simulink model "model"  (R2019a)
settings: Solver=ode113  StartTime=0.0  StopTime=25  RelTol=1e-3
undefined symbols (not defined in the file): sigbuilder_block
libraries: simulink x3
settings Model: Creator=lenovo  LastModifiedBy=FF
settings DataIOCC: ReturnWorkspaceOutputs=off
settings DebuggingCC: ArithmeticOperatorsInVariantConditions=warning
settings SFSimCC: SimUseLocalCustomCode=off
settings RTWCC: RTWUseLocalCustomCode=off

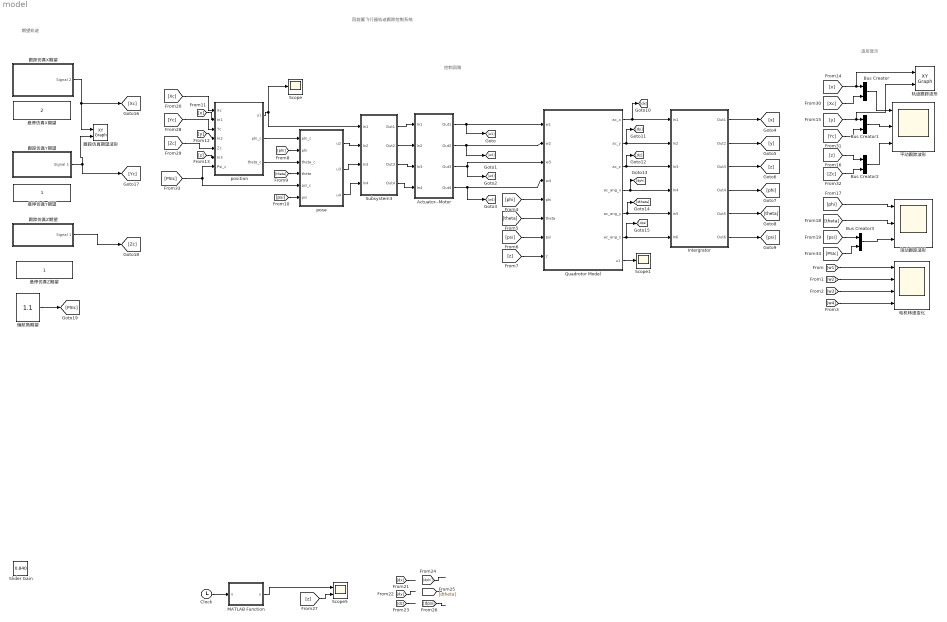
== system model ==
  note: 波形显示
  note: 控制回路
  note: 期望轨迹
  note: 四旋翼飞行器轨迹跟踪控制系统
  Actuator--Motor : Subsystem
  Bus Creator{,1..3} (4 alike) : BusCreator  Inputs=2
  Clock : Clock
  Intergrator : Subsystem
  MATLAB Function : MATLAB Function  TreatAsAtomicUnit=on
  Quadrotor Model : MATLAB Function  TreatAsAtomicUnit=on
  Scope : Scope
  Scope1 : Scope
  Scope5 : Scope  NumInputPorts=2
  Slider Gain : simulink/Math Operations/Slider Gain  gain=0.840  low=0  high=2
  Subsystem3 : Subsystem
  pose : Subsystem
  position : Subsystem
  偏航角期望 : Constant  Value=1.1
  平动跟踪波形 : Scope  NumInputPorts=3
  悬停仿真X期望 : Constant  Value=2
  悬停仿真Y期望 : Constant
  悬停仿真Z期望 : Constant
  滚动跟踪波形 : Scope  NumInputPorts=3
  电机转速变化 : Scope  NumInputPorts=4
  跟踪仿真X期望 : Subsystem  Tag=STV Subsys  LoadFcn=sigbuilder_block('load');  StartFcn=sigbuilder_block('start');  StopFcn=sigbuilder_block('stop');  ClipboardFcn=sigbuilder_block('clipboard');  mask(Sigbuilder block){tuvar=[0:10]}
      mask help: Simulink:masks:SigbuilderBlock_MD
      mask init:
      | if ~strcmp(get_param(bdroot(gcbh),'SimulationStatus'),'stopped') tuvar = sigbuilder_block('maskInit'); end
      settings: CopyFcn=sigbuilder_block('copy');  DeleteFcn=sigbuilder_block('delete');  ModelCloseFcn=sigbuilder_block('modelClose');  PreSaveFcn=sigbuilder_block('preSave');  PauseFcn=sigbuilder_block('pause');  ContinueFcn=sigbuilder_block('continue');  NameChangeFcn=sigbuilder_block('namechange');  OpenFcn=sigbuilder_block('open',[374.4 110.4 550.8 400.2 ]);  CloseFcn=sigbuilder_block('close');
      mask Display: plot(0, 0, 100, 100,[2, 2, 32, 32, 2], [68, 8, 8, 68, 68],[32, 2], [38, 38], [32, 19, 2],[53, 60, 44], [32, 17, 17, 2],[16, 16, 31, 31]);txt = getActiveGroup(gcbh);text(2, 100, txt,'verticalAlignment', 'top');
  跟踪仿真Y期望 : Subsystem  Tag=STV Subsys  LoadFcn=sigbuilder_block('load');  StartFcn=sigbuilder_block('start');  StopFcn=sigbuilder_block('stop');  ClipboardFcn=sigbuilder_block('clipboard');  mask(Sigbuilder block){tuvar=[0:10]}
      mask help: Simulink:masks:SigbuilderBlock_MD
      mask init:
      | if ~strcmp(get_param(bdroot(gcbh),'SimulationStatus'),'stopped') tuvar = sigbuilder_block('maskInit'); end
      settings: CopyFcn=sigbuilder_block('copy');  DeleteFcn=sigbuilder_block('delete');  ModelCloseFcn=sigbuilder_block('modelClose');  PreSaveFcn=sigbuilder_block('preSave');  PauseFcn=sigbuilder_block('pause');  ContinueFcn=sigbuilder_block('continue');  NameChangeFcn=sigbuilder_block('namechange');  OpenFcn=sigbuilder_block('open',[268.8 123 550.8 400.2 ]);  CloseFcn=sigbuilder_block('close');
      mask Display: plot(0, 0, 100, 100,[2, 2, 32, 32, 2], [68, 8, 8, 68, 68],[32, 2], [38, 38], [32, 19, 2],[53, 60, 44], [32, 17, 17, 2],[16, 16, 31, 31]);txt = getActiveGroup(gcbh);text(2, 100, txt,'verticalAlignment', 'top');
  跟踪仿真Z期望 : Subsystem  Tag=STV Subsys  LoadFcn=sigbuilder_block('load');  StartFcn=sigbuilder_block('start');  StopFcn=sigbuilder_block('stop');  ClipboardFcn=sigbuilder_block('clipboard');  mask(Sigbuilder block){tuvar=[0:10]}
      mask help: Simulink:masks:SigbuilderBlock_MD
      mask init:
      | if ~strcmp(get_param(bdroot(gcbh),'SimulationStatus'),'stopped') tuvar = sigbuilder_block('maskInit'); end
      settings: CopyFcn=sigbuilder_block('copy');  DeleteFcn=sigbuilder_block('delete');  ModelCloseFcn=sigbuilder_block('modelClose');  PreSaveFcn=sigbuilder_block('preSave');  PauseFcn=sigbuilder_block('pause');  ContinueFcn=sigbuilder_block('continue');  NameChangeFcn=sigbuilder_block('namechange');  OpenFcn=sigbuilder_block('open',[359.4 96 550.8 400.2 ]);  CloseFcn=sigbuilder_block('close');
      mask Display: plot(0, 0, 100, 100,[2, 2, 32, 32, 2], [68, 8, 8, 68, 68],[32, 2], [38, 38], [32, 19, 2],[53, 60, 44], [32, 17, 17, 2],[16, 16, 31, 31]);txt = getActiveGroup(gcbh);text(2, 100, txt,'verticalAlignment', 'top');
  跟踪仿真期望波形 : simulink/Sinks/XY Graph  xmin=0  xmax=3  ymin=0  ymax=3  st=1
  轨迹跟踪波形 : simulink/Sinks/XY Graph  xmin=0  xmax=3  ymin=0  ymax=3  st=7.5
  wires:
  Quadrotor Model/2(ac_y) -> Intergrator/2(In2), [dy]
  Quadrotor Model/4(ac_ang_x) -> Intergrator/4(In4), [dphi]
  Quadrotor Model/5(ac_ang_y) -> Intergrator/5(In5), [dtheta]
  Quadrotor Model/6(ac_ang_z) -> Intergrator/6(In6), [dpsi]
  Clock/1 -> MATLAB Function/1(u)
  Actuator--Motor/1(Out1) -> Quadrotor Model/1(w1), [w1]
  Actuator--Motor/2(Out2) -> [w2], Quadrotor Model/2(w2)
  Actuator--Motor/3(Out3) -> [w3], Quadrotor Model/3(w3)
  Actuator--Motor/4(Out4) -> Quadrotor Model/4(w4), [w4]
  pose/3(u4) -> Subsystem3/4(In4)
  pose/2(u3) -> Subsystem3/3(In3)
  pose/1(u2) -> Subsystem3/2(In2)
  position/1(u1) -> Scope/1, Subsystem3/1(In1)
  position/3(theta_c) -> pose/3(theta_c)
  position/2(phi_c) -> pose/1(phi_c)
  Quadrotor Model/7(u1) -> Scope1/1
  Subsystem3/1(Out1) -> Actuator--Motor/1(In1)
  Subsystem3/2(Out2) -> Actuator--Motor/2(In2)
  Subsystem3/3(Out3) -> Actuator--Motor/3(In3)
  Subsystem3/4(Out4) -> Actuator--Motor/4(In4)
  Quadrotor Model/1(ac_x) -> Intergrator/1(In1), [dx]
  Quadrotor Model/3(ac_z) -> Intergrator/3(In3), [dz]
  [w1] -> 电机转速变化/1
  [w2] -> 电机转速变化/2
  [w3] -> 电机转速变化/3
  [w4] -> 电机转速变化/4
  Intergrator/1(Out1) -> [x]
  Intergrator/2(Out2) -> [y]
  Intergrator/4(Out4) -> [phi]
  Intergrator/5(Out5) -> [theta]
  Intergrator/6(Out6) -> [psi]
  [phi] -> Quadrotor Model/5(phi)
  [theta] -> Quadrotor Model/6(theta)
  [psi] -> Quadrotor Model/7(psi)
  [z] -> Quadrotor Model/8(z)
  Intergrator/3(Out3) -> [z]
  [phi] -> pose/2(phi)
  [theta] -> pose/4(theta)
  [psi] -> pose/6(psi)
  [x] -> position/2(In1)
  [y] -> position/4(In2)
  [z] -> position/6(In3)
  [x] -> 轨迹跟踪波形/1, Bus Creator/1
  [y] -> Bus Creator1/1, 轨迹跟踪波形/2
  [phi] -> 滚动跟踪波形/1
  [theta] -> 滚动跟踪波形/2
  MATLAB Function/1(y) -> Scope5/1
  [dx] -> ?
  [dy] -> ?
  [dz] -> ?
  [dphi] -> ?
  [dtheta] -> ?
  [dpsi] -> ?
  [z] -> Scope5/2
  跟踪仿真X期望/1(Signal 2) -> 跟踪仿真期望波形/1, [Xc]
  跟踪仿真Y期望/1(Signal 1) -> [Yc], 跟踪仿真期望波形/2
  [Xc] -> position/1(Xc)
  [Yc] -> position/3(Yc)
  [Zc] -> position/5(Zc)
  [Xc] -> Bus Creator/2
  Bus Creator/1 -> 平动跟踪波形/1
  [Yc] -> Bus Creator1/2
  Bus Creator1/1 -> 平动跟踪波形/2
  [z] -> Bus Creator2/1
  [Zc] -> Bus Creator2/2
  Bus Creator2/1 -> 平动跟踪波形/3
  偏航角期望/1 -> [PSIc]
  [PSIc] -> position/7(Psi_c), pose/5(psi_c)
  [psi] -> Bus Creator3/1
  [PSIc] -> Bus Creator3/2
  Bus Creator3/1 -> 滚动跟踪波形/3
  跟踪仿真Z期望/1(Signal 1) -> [Zc]

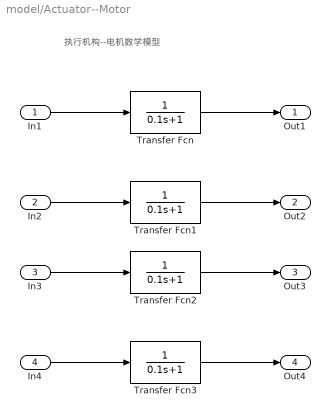
== system model/Actuator--Motor ==
  note: 执行机构--电机数学模型
  In1 : Inport
  In2 : Inport  Port=2
  In3 : Inport  Port=3
  In4 : Inport  Port=4
  Transfer Fcn{,1..3} (4 alike) : TransferFcn  Denominator=[0.1 1]
  Out1 : Outport
  Out2 : Outport  Port=2
  Out3 : Outport  Port=3
  Out4 : Outport  Port=4
  wires:
  In1/1 -> Transfer Fcn/1
  In2/1 -> Transfer Fcn1/1
  In3/1 -> Transfer Fcn2/1
  In4/1 -> Transfer Fcn3/1
  Transfer Fcn/1 -> Out1/1
  Transfer Fcn1/1 -> Out2/1
  Transfer Fcn2/1 -> Out3/1
  Transfer Fcn3/1 -> Out4/1

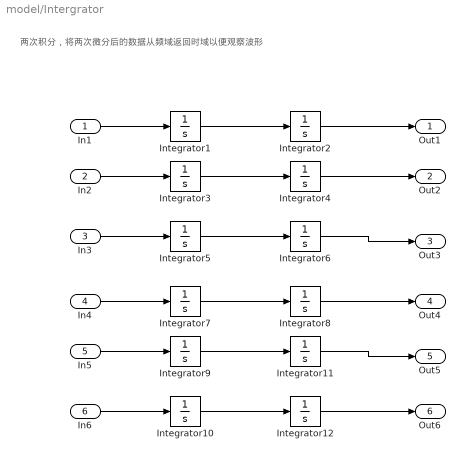
== system model/Intergrator ==
  note: 两次积分，将两次微分后的数据从频域返回时域以便观察波形
  In1 : Inport
  In2 : Inport  Port=2
  In3 : Inport  Port=3
  In4 : Inport  Port=4
  In5 : Inport  Port=5
  In6 : Inport  Port=6
  Integrator{1..12} (12 alike) : Integrator
  Out1 : Outport
  Out2 : Outport  Port=2
  Out3 : Outport  Port=3
  Out4 : Outport  Port=4
  Out5 : Outport  Port=5
  Out6 : Outport  Port=6
  wires:
  Integrator1/1 -> Integrator2/1
  Integrator2/1 -> Out1/1
  In1/1 -> Integrator1/1
  In2/1 -> Integrator3/1
  Integrator3/1 -> Integrator4/1
  Integrator4/1 -> Out2/1
  In3/1 -> Integrator5/1
  Integrator5/1 -> Integrator6/1
  Integrator8/1 -> Out4/1
  Integrator7/1 -> Integrator8/1
  In4/1 -> Integrator7/1
  Integrator11/1 -> Out5/1
  Integrator9/1 -> Integrator11/1
  In5/1 -> Integrator9/1
  Integrator12/1 -> Out6/1
  Integrator10/1 -> Integrator12/1
  In6/1 -> Integrator10/1
  Integrator6/1 -> Out3/1

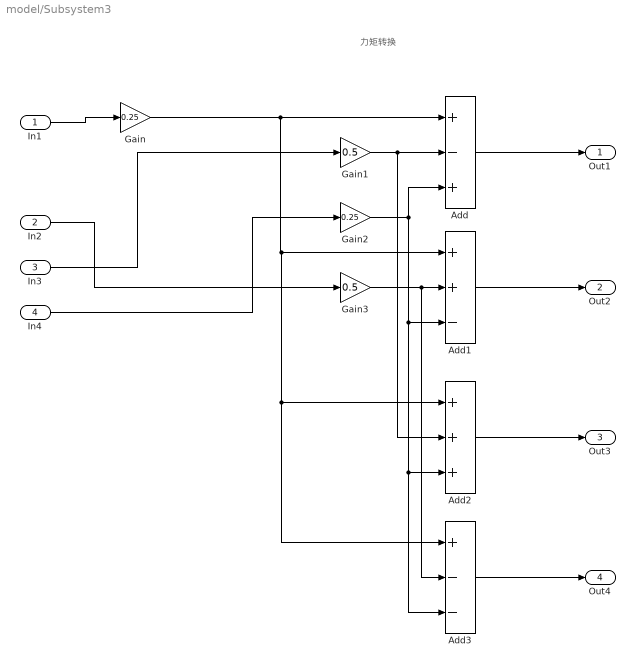
== system model/Subsystem3 ==
  note: 力矩转换
  In1 : Inport
  In2 : Inport  Port=2
  In3 : Inport  Port=3
  In4 : Inport  Port=4
  Add : Sum  Inputs=+-+
  Add1 : Sum  Inputs=++-
  Add2 : Sum  Inputs=+++
  Add3 : Sum  Inputs=+--
  Gain : Gain  Gain=0.25
  Gain1 : Gain  Gain=0.5
  Gain2 : Gain  Gain=0.25
  Gain3 : Gain  Gain=0.5
  Out1 : Outport
  Out2 : Outport  Port=2
  Out3 : Outport  Port=3
  Out4 : Outport  Port=4
  wires:
  In1/1 -> Gain/1
  In2/1 -> Gain3/1
  In4/1 -> Gain2/1
  Add3/1 -> Out4/1
  Add/1 -> Out1/1
  In3/1 -> Gain1/1
  Gain1/1 -> Add2/2, Add/2
  Add2/1 -> Out3/1
  Gain2/1 -> Add/3, Add2/3, Add3/3, Add1/3
  Gain3/1 -> Add3/2, Add1/2
  Add1/1 -> Out2/1
  Gain/1 -> Add3/1, Add2/1, Add1/1, Add/1

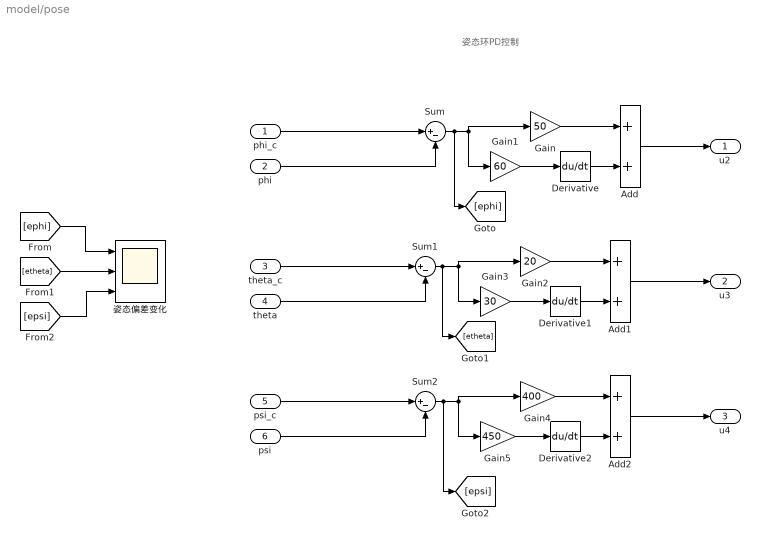
== system model/pose ==
  note: 姿态环PD控制
  phi_c : Inport
  phi : Inport  Port=2
  theta_c : Inport  Port=3
  theta : Inport  Port=4
  psi_c : Inport  Port=5
  psi : Inport  Port=6
  Add : Sum
  Add1 : Sum
  Add2 : Sum
  Derivative : Derivative
  Derivative1 : Derivative
  Derivative2 : Derivative
  Gain : Gain  Gain=50
  Gain1 : Gain  Gain=60
  Gain2 : Gain  Gain=20
  Gain3 : Gain  Gain=30
  Gain4 : Gain  Gain=400
  Gain5 : Gain  Gain=450
  Sum : Sum  Inputs=|+-
  Sum1 : Sum  Inputs=|+-
  Sum2 : Sum  Inputs=|+-
  姿态偏差变化 : Scope  NumInputPorts=3
  u2 : Outport
  u3 : Outport  Port=2
  u4 : Outport  Port=3
  wires:
  phi_c/1 -> Sum/1
  Add/1 -> u2/1
  phi/1 -> Sum/2
  theta/1 -> Sum1/2
  theta_c/1 -> Sum1/1
  Add1/1 -> u3/1
  psi/1 -> Sum2/2
  psi_c/1 -> Sum2/1
  Add2/1 -> u4/1
  Sum/1 -> [ephi], Gain1/1, Gain/1
  Gain1/1 -> Derivative/1
  Gain/1 -> Add/1
  Derivative/1 -> Add/2
  Sum1/1 -> [etheta], Gain3/1, Gain2/1
  Gain2/1 -> Add1/1
  Derivative1/1 -> Add1/2
  Gain3/1 -> Derivative1/1
  Sum2/1 -> [epsi], Gain5/1, Gain4/1
  Gain4/1 -> Add2/1
  Gain5/1 -> Derivative2/1
  Derivative2/1 -> Add2/2
  [ephi] -> 姿态偏差变化/1
  [etheta] -> 姿态偏差变化/2
  [epsi] -> 姿态偏差变化/3

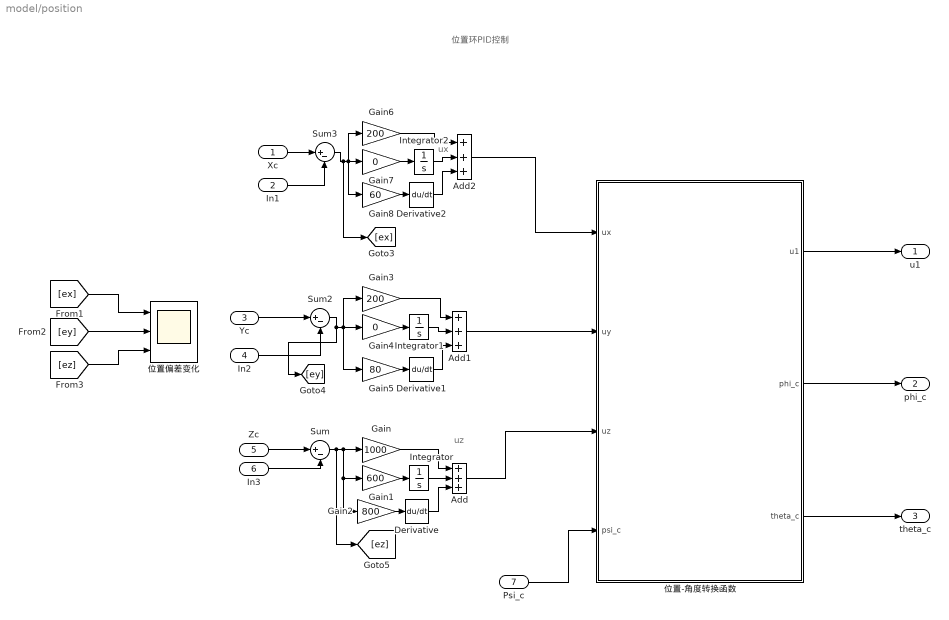
== system model/position ==
  note: 位置环PID控制
  note: uz
  note: ux
  Xc : Inport
  In1 : Inport  Port=2
  Yc : Inport  Port=3
  In2 : Inport  Port=4
  Zc : Inport  Port=5
  In3 : Inport  Port=6
  Psi_c : Inport  Port=7
  Add : Sum  Inputs=+++
  Add1 : Sum  Inputs=+++
  Add2 : Sum  Inputs=+++
  Derivative : Derivative
  Derivative1 : Derivative
  Derivative2 : Derivative
  Gain : Gain  Gain=1000
  Gain1 : Gain  Gain=600
  Gain2 : Gain  Gain=800
  Gain3 : Gain  Gain=200
  Gain4 : Gain  Gain=0
  Gain5 : Gain  Gain=80
  Gain6 : Gain  Gain=200
  Gain7 : Gain  Gain=0
  Gain8 : Gain  Gain=60
  Integrator : Integrator
  Integrator1 : Integrator
  Integrator2 : Integrator
  Sum : Sum  Inputs=|+-
  Sum2 : Sum  Inputs=|+-
  Sum3 : Sum  Inputs=|+-
  位置-角度转换函数 : MATLAB Function  TreatAsAtomicUnit=on
  位置偏差变化 : Scope  NumInputPorts=3
  u1 : Outport
  phi_c : Outport  Port=2
  theta_c : Outport  Port=3
  wires:
  Xc/1 -> Sum3/1
  Yc/1 -> Sum2/1
  In1/1 -> Sum3/2
  In2/1 -> Sum2/2
  Psi_c/1 -> 位置-角度转换函数/4(psi_c)
  位置-角度转换函数/1(u1) -> u1/1
  位置-角度转换函数/2(phi_c) -> phi_c/1
  位置-角度转换函数/3(theta_c) -> theta_c/1
  Gain1/1 -> Integrator/1
  Gain2/1 -> Derivative/1
  Sum/1 -> [ez], Gain/1, Gain1/1, Gain2/1
  Gain/1 -> Add/1
  Integrator/1 -> Add/2
  Derivative/1 -> Add/3
  In3/1 -> Sum/2
  Derivative1/1 -> Add1/3
  Gain3/1 -> Add1/1
  Integrator1/1 -> Add1/2
  Sum2/1 -> [ey], Gain4/1, Gain5/1, Gain3/1
  Gain4/1 -> Integrator1/1
  Gain5/1 -> Derivative1/1
  Gain7/1 -> Integrator2/1
  Derivative2/1 -> Add2/3
  Integrator2/1 -> Add2/2
  Gain6/1 -> Add2/1
  Gain8/1 -> Derivative2/1
  Sum3/1 -> [ex], Gain7/1, Gain8/1, Gain6/1
  Add2/1 -> 位置-角度转换函数/1(ux)
  Add1/1 -> 位置-角度转换函数/2(uy)
  Add/1 -> 位置-角度转换函数/3(uz)
  [ex] -> 位置偏差变化/1
  [ey] -> 位置偏差变化/2
  [ez] -> 位置偏差变化/3
  Zc/1 -> Sum/1

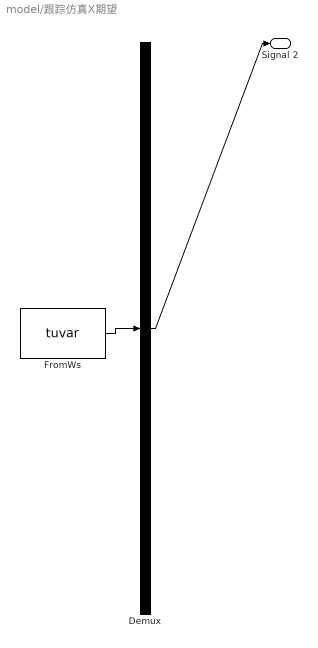
== system model/跟踪仿真X期望 ==
  Demux : Demux  Tag=STV Demux  Outputs=1
  FromWs : FromWorkspace  Tag=STV FromWs  VariableName=tuvar  SampleTime=0
      SigBuilderData=|
      | common.afterFinalStr = 'Extrapolate'
      | common.sampleTime = 0
      | dataSet.timeRange = [0 30]
      | dataSet.name = 'Group 1'
      | sbobj.Groups.Name = 'Group 1'
      | sbobj.Groups.Signals.Name = 'Signal 2'
      | sbobj.Groups.Signals.XData = [0 3 3 10 10 16 16 30]
      | sbobj.Groups.Signals.YData = [0 0 1 1 2 2 3 3]
      | sbobj.Groups.TimeRange = [0 30]
  Signal 2 : Outport  Tag=STV Outport
  wires:
  FromWs/1 -> Demux/1
  Demux/1 -> Signal 2/1

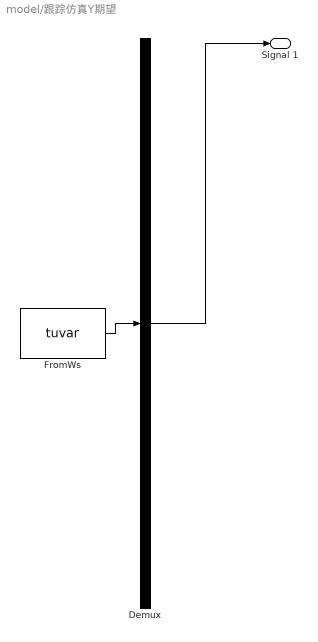
== system model/跟踪仿真Y期望 ==
  Demux : Demux  Tag=STV Demux  Outputs=1
  FromWs : FromWorkspace  Tag=STV FromWs  VariableName=tuvar  SampleTime=0
      SigBuilderData=|
      | common.afterFinalStr = 'Extrapolate'
      | common.sampleTime = 0
      | dataSet.timeRange = [0 30]
      | dataSet.name = 'Group 1'
      | sbobj.Groups.Name = 'Group 1'
      | sbobj.Groups.Signals.Name = 'Signal 1'
      | sbobj.Groups.Signals.XData = [0 3 3 10 16 16 30]
      | sbobj.Groups.Signals.YData = [0 0 1 1 1 1.5 1.5]
      | sbobj.Groups.TimeRange = [0 30]
  Signal 1 : Outport  Tag=STV Outport
  wires:
  Demux/1 -> Signal 1/1
  FromWs/1 -> Demux/1

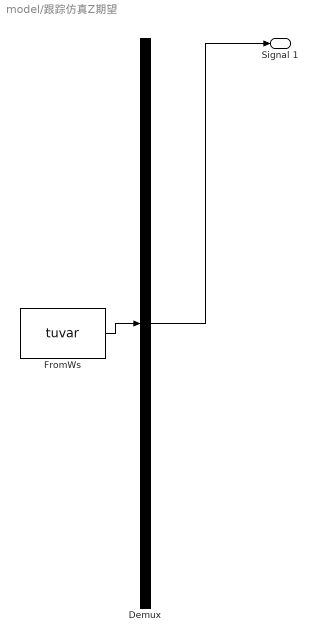
== system model/跟踪仿真Z期望 ==
  Demux : Demux  Tag=STV Demux  Outputs=1
  FromWs : FromWorkspace  Tag=STV FromWs  VariableName=tuvar  SampleTime=0
      SigBuilderData=|
      | common.afterFinalStr = 'Extrapolate'
      | common.sampleTime = 0
      | dataSet.timeRange = [0 10]
      | dataSet.name = 'Group 1'
      | sbobj.Groups.Name = 'Group 1'
      | sbobj.Groups.Signals.Name = 'Signal 1'
      | sbobj.Groups.Signals.XData = [0 3 3 8 10]
      | sbobj.Groups.Signals.YData = [0 0 0.4 0.4 0.4]
  Signal 1 : Outport  Tag=STV Outport
  wires:
  Demux/1 -> Signal 1/1
  FromWs/1 -> Demux/1

== matlab function model/position/位置-角度转换函数 ==
  data: ux input; u1 output; uy input; uz input; psi_c input; phi_c output; theta_c output
%位置-姿态角度转换函数
function [u1,phi_c,theta_c] = fcn(ux,uy,uz,psi_c)
m=1.2;g=9.8;
u1=m*sqrt(ux^2+uy^2+(uz+g)^2);
phi_c=asin(m/u1*(ux*sin(psi_c)-uy*cos(psi_c)));
theta_c=atan((ux*cos(psi_c)+uy*sin(psi_c))/(uz+g));


%theta_c=asin((ux*m-u1*sin(psi_c)*sin(phi_c))/(u1*cos(psi_c)*cos(phi_c)));

== matlab function model/Quadrotor Model ==
  data: w1 input; ac_x output; ac_y output; ac_z output; w2 input; w3 input; w4 input; phi input; theta input; psi input; ac_ang_x output; ac_ang_y output; ac_ang_z output; u1 output; z input
%被控对象--四旋翼飞行器数学模型
function [ac_x,ac_y,ac_z,ac_ang_x,ac_ang_y,ac_ang_z,u1 ] = fcn(w1,w2,w3,w4,phi,theta,psi,z)
%根据参考资料，定义所需参数 
kt=3.13e-5;kd=7.5e-7;Ix=0.0197;Iy=0.0197;Iz=0.0393;m=1.2;g=9.8;l=0.25;
u1=kt*(w1^2+w2^2+w3^2+w4^2);
u2=kt*(w2^2-w4^2);
u3=kt*(w3^2-w1^2);
u4=kd*(w1^2+w3^2-w2^2-w4^2);
if u1<=m*g && z==0
    a1=g-cos(phi)*cos(theta)*u1/m;
else
    a1=0;
end
ac_x=(cos(psi)*sin(theta)*cos(phi)+sin(phi)*sin(psi))*u1/m;
ac_y=(sin(psi)*sin(theta)*cos(phi)-cos(psi)*sin(phi))*u1/m;
ac_z=cos(phi)*cos(theta)*u1/m-g+a1;
ac_ang_x=l*u2/Ix;
ac_ang_y=l*u3/Iy;
ac_ang_z=l*u4/Iz;

== matlab function model/MATLAB Function ==
  data: u input; y output
function y = fcn(u)

y = 0.2*u;
